simulink model "Schemat_ADRC_manipulator"  (R2024a)
settings: Solver=ode1be  StartTime=0.0  StopTime=10.0  FixedStep=0.01  MaxStep=0.01  MinStep=0.001  RelTol=1e-3
libraries: adrc_toolbox_library x1, slpidlib x1
settings Model: Creator=janek  LastModifiedBy=janek
settings SolverCC: InitialStep=0.005  ShapePreserveControl=EnableAll

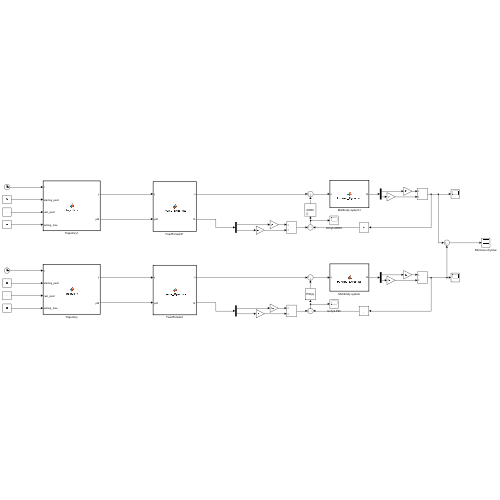
[thumbnail: Simulink's stored preview of the top-level diagram]
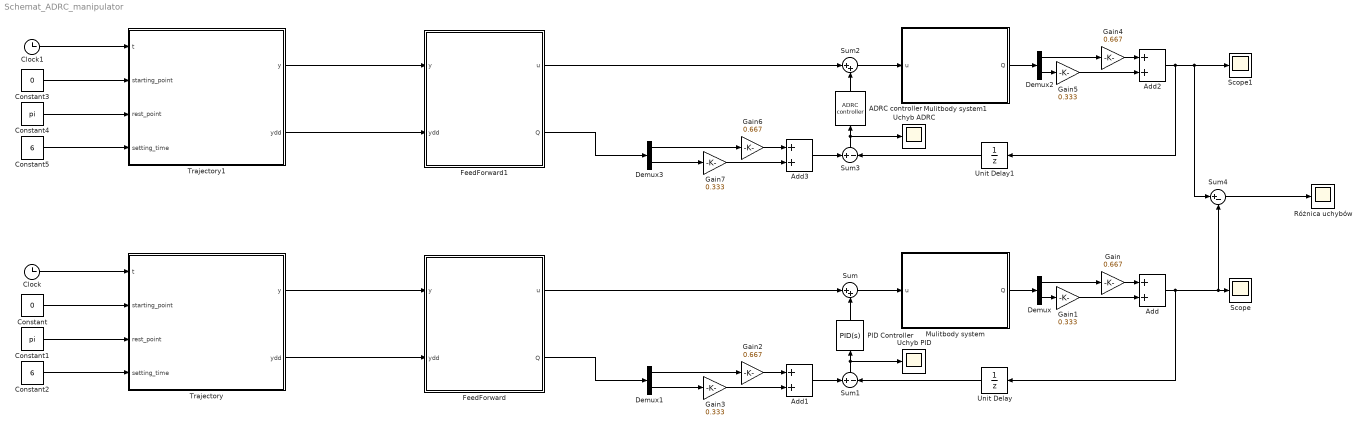
== system Schemat_ADRC_manipulator ==
  ADRC controller : adrc_toolbox_library/ADRC controller  dynamicsOrder=2  inputGainParameter=0.1  inputGainSource=Internal  observerBandwidth=50  observerBandwidthSource=Internal  controllerBandwidth=10  controllerBandwidthSource=Internal  saturationEnabled=off  UpperLimit=10  LowerLimit=-10  deadTimeEnabled=off  deadTime=0.2  observerOutputEnabled=off  observerOutputChoice=Estimated total disturbance
      settings: SourceProductName=ADRC Toolbox
  Add{,1..3} (4 alike) : Sum
  Clock : Clock
  Clock1 : Clock
  Constant : Constant  Value=0
  Constant1 : Constant  Value=pi
  Constant2 : Constant  Value=6
  Constant3 : Constant  Value=0
  Constant4 : Constant  Value=pi
  Constant5 : Constant  Value=6
  Demux{,1..3} (4 alike) : Demux  Outputs=2
  FeedForward : MATLAB Function  TreatAsAtomicUnit=on
  FeedForward1 : MATLAB Function  TreatAsAtomicUnit=on
  Gain{,2,4,6} (4 alike) : Gain  Gain=0.667
  Gain{1,3,5,7} (4 alike) : Gain  Gain=0.333
  Mulitbody system : MATLAB Function  TreatAsAtomicUnit=on
  Mulitbody system1 : MATLAB Function  TreatAsAtomicUnit=on
  PID Controller : slpidlib/PID Controller  Controller=PID  Form=Parallel  TimeDomain=Continuous-time  UseExternalTs=off  SampleTime=-1  IntegratorMethod=Forward Euler  FilterMethod=Forward Euler  ControllerParametersSource=internal  P=200  I=3  UseKiTs=off  D=160  UseExternalDerivativeSource=off  N=100  UseFilter=on  TunerSelectOption=Transfer Function Based (PID Tuner App)  InitialConditionSource=internal  InitialConditionForIntegrator=0  InitialConditionForFilter=0  DifferentiatorICPrevScaledInput=0  ExternalReset=none  TrackingMode=off  Kt=1  LimitOutput=off  SatLimitsSource=internal  UpperSaturationLimit=inf  LowerSaturationLimit=-inf  LinearizeAsGain=on  AntiWindupMode=none  Kb=1  LimitIntegrator=off  UpperIntegratorSaturationLimit=inf  LowerIntegratorSaturationLimit=-inf  POutMin=[]  POutMax=[]  IOutMin=[]  IOutMax=[]  DOutMin=[]  DOutMax=[]  NOutMin=[]  NOutMax=[]  SumOutMin=[]  SumOutMax=[]  SaturationOutMin=[]  SaturationOutMax=[]  PParamMin=[]  PParamMax=[]  IParamMin=[]  IParamMax=[]  DParamMin=[]  DParamMax=[]  NParamMin=[]  NParamMax=[]  KbParamMin=[]  KbParamMax=[]  KtParamMin=[]  KtParamMax=[]  KbOutMin=[]  KbOutMax=[]  KtOutMin=[]  KtOutMax=[]  IntegratorOutMin=[]  IntegratorOutMax=[]  FilterOutMin=[]  FilterOutMax=[]  SumI1OutMin=[]  SumI1OutMax=[]  SumI2OutMin=[]  SumI2OutMax=[]  SumI3OutMin=[]  SumI3OutMax=[]  SumI4OutMin=[]  SumI4OutMax=[]  SumDOutMin=[]  SumDOutMax=[]  DifferentiatorOutMin=[]  DifferentiatorOutMax=[]  FilterDiffOutCoefMin=[]  FilterDiffOutCoefMax=[]  ReciprocalOutMin=[]  ReciprocalOutMax=[]  SumDenOutMin=[]  SumDenOutMax=[]  SumNumOutMin=[]  SumNumOutMax=[]  DivideOutMin=[]  DivideOutMax=[]  UdiffTsProdOutMin=[]  UdiffTsProdOutMax=[]  NTsProdOutMin=[]  NTsProdOutMax=[]  UintegralTsProdOutMin=[]  UintegralTsProdOutMax=[]  UngainTsProdOutMin=[]  UngainTsProdOutMax=[]  ClampingZeroOutDataTypeStr=Inherit: Inherit via back propagation  ClampingZeroOutMin=[]  ClampingZeroOutMax=[]  FilterDenConstantOutDataTypeStr=Inherit: Inherit via back propagation  FilterDenConstantOutMin=[]  FilterDenConstantOutMax=[]  PCopyOutDataTypeStr=Inherit: Inherit via back propagation  PCopyOutMin=[]  PCopyOutMax=[]  NCopyOutDataTypeStr=Inherit: Inherit via back propagation  NCopyOutMin=[]  NCopyOutMax=[]  IntegratorContinuousStateAttributes=''  IntegratorStateMustResolveToSignalObject=off  IntegratorRTWStateStorageClass=Auto  FilterContinuousStateAttributes=''  FilterStateMustResolveToSignalObject=off  FilterRTWStateStorageClass=Auto  ParallelPVariant=InternalParameters  IdealPVariant=Disabled  IVariant=InternalParameters  DVariant=InternalParameters  IntegratorVariant=Continuous  SatVariant=Disabled  AWVariant=Passthrough  PCopyVariant=Disabled  TRVariant=Disabled  FdbkBlocksVariant=Forward  IdealPFdbkVariant=Disabled  SatFdbkVariant=Disabled  DerivativeFilterVariant=ContFilter  NVariant=InternalParameters  NCopyVariant=Disabled  FilterICVariant=InternalICsFilter  IntegratorICVariant=InternalICs  ExternalResetVariant=Disabled  TRSumVariant=Passthrough  SumFdbkVariant=Disabled  SumVariant=Sum_PID  TsampFilterVariant=InternalTs  TsampNgainVariant=Passthrough  TsampIntegralVariant=Disabled_SignalSpec  ExternalSaturationOutDataTypeStr=Inherit: Same as second input  DerivativeSourceVariant=ErrorSignal
  Różnica uchybów : Scope
  Scope : Scope
  Scope1 : Scope
  Sum : Sum  Inputs=|++
  Sum1 : Sum  Inputs=+|-
  Sum2 : Sum  Inputs=|++
  Sum3 : Sum  Inputs=+|-
  Sum4 : Sum  Inputs=|+-
  Trajectory : MATLAB Function  TreatAsAtomicUnit=on
  Trajectory1 : MATLAB Function  TreatAsAtomicUnit=on
  Uchyb ADRC : Scope
  Uchyb PID : Scope
  Unit Delay : UnitDelay  SampleTime=-1  HasFrameUpgradeWarning=on
  Unit Delay1 : UnitDelay  SampleTime=-1  HasFrameUpgradeWarning=on
  wires:
  Clock/1 -> Trajectory/1(t)
  Constant/1 -> Trajectory/2(starting_point)
  Constant1/1 -> Trajectory/3(rest_point)
  Constant2/1 -> Trajectory/4(setting_time)
  Trajectory/1(y) -> FeedForward/1(y)
  Trajectory/2(ydd) -> FeedForward/2(ydd)
  Mulitbody system/1(Q) -> Demux/1
  Demux/1 -> Gain/1
  Demux/2 -> Gain1/1
  Gain/1 -> Add/1
  Gain1/1 -> Add/2
  Add/1 -> Sum4/2, Scope/1, Unit Delay/1
  FeedForward/1(u) -> Sum/1
  Sum/1 -> Mulitbody system/1(u)
  PID Controller/1 -> Sum/2
  Sum1/1 -> Uchyb PID/1, PID Controller/1
  FeedForward/2(Q) -> Demux1/1
  Add1/1 -> Sum1/1
  Gain2/1 -> Add1/1
  Gain3/1 -> Add1/2
  Demux1/2 -> Gain3/1
  Demux1/1 -> Gain2/1
  Unit Delay/1 -> Sum1/2
  Sum3/1 -> Uchyb ADRC/1, ADRC controller/1
  Add3/1 -> Sum3/1
  Gain6/1 -> Add3/1
  Gain7/1 -> Add3/2
  FeedForward1/2(Q) -> Demux3/1
  Demux3/1 -> Gain6/1
  ADRC controller/1 -> Sum2/2
  Sum2/1 -> Mulitbody system1/1(u)
  FeedForward1/1(u) -> Sum2/1
  Demux3/2 -> Gain7/1
  Mulitbody system1/1(Q) -> Demux2/1
  Gain4/1 -> Add2/1
  Add2/1 -> Sum4/1, Scope1/1, Unit Delay1/1
  Unit Delay1/1 -> Sum3/2
  Trajectory1/2(ydd) -> FeedForward1/2(ydd)
  Constant5/1 -> Trajectory1/4(setting_time)
  Constant4/1 -> Trajectory1/3(rest_point)
  Gain5/1 -> Add2/2
  Trajectory1/1(y) -> FeedForward1/1(y)
  Constant3/1 -> Trajectory1/2(starting_point)
  Clock1/1 -> Trajectory1/1(t)
  Demux2/2 -> Gain5/1
  Demux2/1 -> Gain4/1
  Sum4/1 -> Różnica uchybów/1

== matlab function Schemat_ADRC_manipulator/FeedForward ==
  settings: updateMethod=DISCRETE
  data: u output; Q output; y input; ydd input
function [u, Q] = Inverse_Dynamics(y, ydd)
    % Define output sizes for Simulink
    Q = zeros(2, 1); % Ensure Q is a 2x1 vector
    V = zeros(2, 1); % Ensure V is a 2x1 vector
    u = zeros(1, 1); % Ensure u is a scalar
    
    % Declare persistent variables for initial guesses
    persistent initial_guess;
    
    if isempty(initial_guess)
        % Initialize at first call
        initial_guess = [0, 0, 0, 0, 0]; % [q1, q2, v1, v2, u]
    end
    
    % Define parameters
    l1 = 1;
    l2 = 1;
    m1 = 2;
    m2 = 2;
    c = 1;
    d = 0.2;
    J1 = m1 * l1^2 / 12;
    J2 = m2 * l2^2 / 12;
    s1 = l1 / 2;
    s2 = l2 / 2;
    n = 2;
    m = 1;

    % Define functions for M, k, g, and B
    M = @(q)[J1 + m1 * s1^2 + m2 * l1^2, m2 * s2 * l1 * cos(q(2) - q(1));
             m2 * s2 * l1 * cos(q(2) - q(1)), J2 + m2 * s2^2];
    k = @(q, v)[-m2 * s2 * l1 * v(2)^2 * sin(q(2) - q(1)); 
                m2 * s2 * l1 * v(1)^2 * sin(q(2) - q(1))];
    g = @(q, v)[c * (q(2) - q(1)) + d * (v(2) - v(1)); 
               -c * (q(2) - q(1)) - d * (v(2) - v(1))];
    B = [1; 0];
    
    % Optimization options
    options = optimoptions('fsolve', 'Display', 'none', 'Algorithm', 'levenberg-marquardt');
    
    % Function for fsolve
    func = @(unknowns) Inverse_Dynamics_v2(unknowns, M(initial_guess(1:n)), g(initial_guess(1:n), initial_guess(n+1:2*n)),k(initial_guess(1:n), initial_guess(n+1:2*n)), B, y, ydd, initial_guess(1:n)', initial_guess(n+1:2*n)');

    % Solve for the unknowns
    solution = fsolve(func, initial_guess, options);
    initial_guess = solution; % Update the guess for the next call
    
    % Extract results
    u = solution(5);
    Q = solution(1:2)';
    V = solution(3:4)';
end

function Solution = Inverse_Dynamics_v2(unknowns, M, g, k, B, y, ydd, q, v)
    dt = 0.01;
    Q = unknowns(1:2)';
    V = unknowns(3:4)';
    u = unknowns(5);

    % Trajectory defined
    kappa = 0.333;
    phi = Q(1) * (1 - kappa) + Q(2) * kappa - y;
    H = [(1-kappa), kappa];
    Hd = [0, 0];
    h = Hd * V;
    
    % G calculation
    if(H(2) == 0)
    G = [0 1]';
        elseif(H(1) == 0 && H(2) == 1)
    G = [1, 0]';
        else
    G = [1, (-H(2)^(-1) * H(1))]';  
    end
   
      Solution = [(Q - q)/dt - V;
                G'*M * (V - v)/dt - G'*(g-k) - G'*B*u;
                H*inv(M) * (g-k) + H*inv(M)*B*u + h - ydd;
                phi];
end

== matlab function Schemat_ADRC_manipulator/Trajectory ==
  data: t input; y output; starting_point input; rest_point input; setting_time input; ydd output
function [y, ydd] = Trajectory(t, starting_point, rest_point, setting_time)
y = starting_point + (rest_point - starting_point)*((126*t^5)/setting_time^5 - (420*t^6)/setting_time^6 + (540*t^7)/setting_time.^7 - (315*t^8)/setting_time^8 + (70*t^9)/setting_time^9);
ydd = (rest_point - starting_point)*((2520*t^3)/setting_time^5 - (12600*t^4)/setting_time^6 + (22680*t^5)/setting_time^7 - (17640*t^6)/setting_time^8 + (5040*t^7)/setting_time^9);

if t > setting_time
    y = rest_point;
    yd = 0;
    ydd = 0;
end
end

== matlab function Schemat_ADRC_manipulator/Mulitbody system ==
  settings: updateMethod=DISCRETE
  data: u input; Q output
function Q  = Forward_Dynamics(u)
    
    % Declare persistent variables for initial guesses
    persistent initial_guess;
    
    if isempty(initial_guess)
        % Initialize at first call
        initial_guess = [0, 0; 0, 0]; 
    end
    q = initial_guess(1:2)';
    v = initial_guess(3:4)';
    l1 = 1;
    l2 = 1;
    m1 = 2;
    m2 = 2;
    c = 1;
    d = 0.2;
    J1 = m1 * l1^2 / 12;
    J2 = m2 * l2^2 / 12;
    s1 = l1 / 2;
    s2 = l2 / 2;

    % Define functions for M, k, g, and B
    M = @(q)1.1*[J1 + m1 * s1^2 + m2 * l1^2, m2 * s2 * l1 * cos(q(2) - q(1));
             m2 * s2 * l1 * cos(q(2) - q(1)), J2 + m2 * s2^2];
    k = @(q, v)[-m2 * s2 * l1 * v(2)^2 * sin(q(2) - q(1)); 
                m2 * s2 * l1 * v(1)^2 * sin(q(2) - q(1))];
    g = @(q, v)[c * (q(2) - q(1)) + d * (v(2) - v(1)); 
               -c * (q(2) - q(1)) - d * (v(2) - v(1))];
    B = [1; 0];

    dt = 0.01;
    a = M(q)\(g(q,v)+B*u -k(q,v));
    V = v + dt * a;
    Q = q + dt * V; 
    initial_guess = [Q,V];
y = u;

== matlab function Schemat_ADRC_manipulator/FeedForward1 ==
  settings: updateMethod=DISCRETE
  data: u output; Q output; y input; ydd input
function [u, Q] = Inverse_Dynamics(y, ydd)
    % Define output sizes for Simulink
    Q = zeros(2, 1); % Ensure Q is a 2x1 vector
    V = zeros(2, 1); % Ensure V is a 2x1 vector
    u = zeros(1, 1); % Ensure u is a scalar
    
    % Declare persistent variables for initial guesses
    persistent initial_guess;
    
    if isempty(initial_guess)
        % Initialize at first call
        initial_guess = [0, 0, 0, 0, 0]; % [q1, q2, v1, v2, u]
    end
    
    % Define parameters
    l1 = 1;
    l2 = 1;
    m1 = 2;
    m2 = 2;
    c = 1;
    d = 0.2;
    J1 = m1 * l1^2 / 12;
    J2 = m2 * l2^2 / 12;
    s1 = l1 / 2;
    s2 = l2 / 2;
    n = 2;
    m = 1;

    % Define functions for M, k, g, and B
    M = @(q)[J1 + m1 * s1^2 + m2 * l1^2, m2 * s2 * l1 * cos(q(2) - q(1));
             m2 * s2 * l1 * cos(q(2) - q(1)), J2 + m2 * s2^2];
    k = @(q, v)[-m2 * s2 * l1 * v(2)^2 * sin(q(2) - q(1)); 
                m2 * s2 * l1 * v(1)^2 * sin(q(2) - q(1))];
    g = @(q, v)[c * (q(2) - q(1)) + d * (v(2) - v(1)); 
               -c * (q(2) - q(1)) - d * (v(2) - v(1))];
    B = [1; 0];
    
    % Optimization options
    options = optimoptions('fsolve', 'Display', 'none', 'Algorithm', 'levenberg-marquardt');
    
    % Function for fsolve
    func = @(unknowns) Inverse_Dynamics_v2(unknowns, M(initial_guess(1:n)), g(initial_guess(1:n), initial_guess(n+1:2*n)),k(initial_guess(1:n), initial_guess(n+1:2*n)), B, y, ydd, initial_guess(1:n)', initial_guess(n+1:2*n)');

    % Solve for the unknowns
    solution = fsolve(func, initial_guess, options);
    initial_guess = solution; % Update the guess for the next call
    
    % Extract results
    u = solution(5);
    Q = solution(1:2)';
    V = solution(3:4)';
end

function Solution = Inverse_Dynamics_v2(unknowns, M, g, k, B, y, ydd, q, v)
    dt = 0.01;
    Q = unknowns(1:2)';
    V = unknowns(3:4)';
    u = unknowns(5);

    % Trajectory defined
    kappa = 0.333;
    phi = Q(1) * (1 - kappa) + Q(2) * kappa - y;
    H = [(1-kappa), kappa];
    Hd = [0, 0];
    h = Hd * V;
    
    % G calculation
    if(H(2) == 0)
    G = [0 1]';
        elseif(H(1) == 0 && H(2) == 1)
    G = [1, 0]';
        else
    G = [1, (-H(2)^(-1) * H(1))]';  
    end
   
      Solution = [(Q - q)/dt - V;
                G'*M * (V - v)/dt - G'*(g-k) - G'*B*u;
                H*inv(M) * (g-k) + H*inv(M)*B*u + h - ydd;
                phi];
end

== matlab function Schemat_ADRC_manipulator/Mulitbody system1 ==
  settings: updateMethod=DISCRETE
  data: u input; Q output
function Q  = Forward_Dynamics(u)
    
    % Declare persistent variables for initial guesses
    persistent initial_guess;
    
    if isempty(initial_guess)
        % Initialize at first call
        initial_guess = [0, 0; 0, 0]; 
    end
    q = initial_guess(1:2)';
    v = initial_guess(3:4)';
    l1 = 1;
    l2 = 1;
    m1 = 2;
    m2 = 2;
    c = 1;
    d = 0.2;
    J1 = m1 * l1^2 / 12;
    J2 = m2 * l2^2 / 12;
    s1 = l1 / 2;
    s2 = l2 / 2;

    % Define functions for M, k, g, and B
    M = @(q)1.1*[J1 + m1 * s1^2 + m2 * l1^2, m2 * s2 * l1 * cos(q(2) - q(1));
             m2 * s2 * l1 * cos(q(2) - q(1)), J2 + m2 * s2^2];
    k = @(q, v)[-m2 * s2 * l1 * v(2)^2 * sin(q(2) - q(1)); 
                m2 * s2 * l1 * v(1)^2 * sin(q(2) - q(1))];
    g = @(q, v)[c * (q(2) - q(1)) + d * (v(2) - v(1)); 
               -c * (q(2) - q(1)) - d * (v(2) - v(1))];
    B = [1; 0];

    dt = 0.01;
    a = M(q)\(g(q,v)+B*u -k(q,v));
    V = v + dt * a;
    Q = q + dt * V; 
    initial_guess = [Q,V];
y = u;

== matlab function Schemat_ADRC_manipulator/Trajectory1 ==
  data: t input; y output; starting_point input; rest_point input; setting_time input; ydd output
function [y, ydd] = Trajectory(t, starting_point, rest_point, setting_time)
y = starting_point + (rest_point - starting_point)*((126*t^5)/setting_time^5 - (420*t^6)/setting_time^6 + (540*t^7)/setting_time.^7 - (315*t^8)/setting_time^8 + (70*t^9)/setting_time^9);
ydd = (rest_point - starting_point)*((2520*t^3)/setting_time^5 - (12600*t^4)/setting_time^6 + (22680*t^5)/setting_time^7 - (17640*t^6)/setting_time^8 + (5040*t^7)/setting_time^9);

if t > setting_time
    y = rest_point;
    yd = 0;
    ydd = 0;
end
end
